simulink model "bh_2dof_compare_models"  (R2017a)
settings: Solver=ode45  StartTime=0.0  StopTime=20  RelTol=1e-5  EnableMultiTasking=on
PreLoadFcn:
  | bh_script_2dof_params
values from neighbouring files (symbols this model uses):
  c1 = 20    [bh_2dof_MATLAB_analysis.m]
  c2 = 50    [bh_2dof_MATLAB_analysis.m]
  c3 = 10    [bh_2dof_MATLAB_analysis.m]
  k1 = 1000    [bh_2dof_MATLAB_analysis.m]
  k2 = 500    [bh_2dof_MATLAB_analysis.m]
  k3 = 100    [bh_2dof_MATLAB_analysis.m]
  m1 = 10    [bh_2dof_MATLAB_analysis.m]
  m2 = 1    [bh_2dof_MATLAB_analysis.m]
undefined symbols (not defined in the file or in its folder): init_x1, init_x1dot, init_x2, init_x2dot
libraries: fl_lib x18, nesl_utility x7
settings Model: Creator=bhorton  LastModifiedBy=bhorton
settings OptimizationCC: LifeSpan=inf
settings DebuggingCC: SFUnexpectedBacktrackingDiag=warning  SFNoUnconditionalDefaultTransitionDiag=warning  SFExecutionAtInitializationDiag=none
settings GRTTargetCC: TargetLangStandard=C89/C90 (ANSI)  GeneratePreprocessorConditionals=Disable all
settings ConfigComp: CovMetricSettings=dw  CovHtmlReporting=on  CovSaveCumulativeToWorkspaceVar=on  CovSaveSingleToWorkspaceVar=on  CovExternalEMLEnable=off

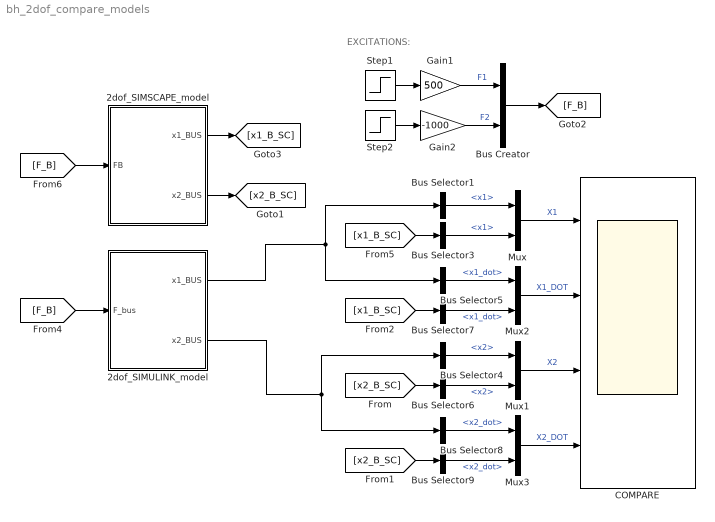
== system bh_2dof_compare_models ==
  note: EXCITATIONS:
  2dof_SIMSCAPE_model : Subsystem
  2dof_SIMULINK_model : Subsystem
  Bus Creator : BusCreator  Inputs=2
  Bus Selector1 : BusSelector  OutputSignals=x1
  Bus Selector3 : BusSelector  OutputSignals=x1
  Bus Selector4 : BusSelector  OutputSignals=x2
  Bus Selector5 : BusSelector  OutputSignals=x1_dot
  Bus Selector6 : BusSelector  OutputSignals=x2
  Bus Selector7 : BusSelector  OutputSignals=x1_dot
  Bus Selector8 : BusSelector  OutputSignals=x2_dot
  Bus Selector9 : BusSelector  OutputSignals=x2_dot
  COMPARE : Scope  NumInputPorts=4
  Gain1 : Gain  Gain=500
  Gain2 : Gain  Gain=-1000
  Mux{,1..3} (4 alike) : Mux  Inputs=2
  Step1 : Step  Time=5  SampleTime=0
  Step2 : Step  Time=10  SampleTime=0
  wires:
  Step1/1 -> Gain1/1
  Gain1/1 -> Bus Creator/1  "F1"
  Step2/1 -> Gain2/1
  Gain2/1 -> Bus Creator/2  "F2"
  Bus Creator/1 -> [F_B]
  [F_B] -> 2dof_SIMSCAPE_model/1(FB)
  [x2_B_SC] -> Bus Selector6/1
  Bus Selector1/1 -> Mux/1  "<x1>"
  [x1_B_SC] -> Bus Selector3/1
  Bus Selector3/1 -> Mux/2  "<x1>"
  Mux/1 -> COMPARE/1  "X1"
  Bus Selector4/1 -> Mux1/1  "<x2>"
  Bus Selector6/1 -> Mux1/2  "<x2>"
  Mux1/1 -> COMPARE/3  "X2"
  2dof_SIMULINK_model/1(x1_BUS) -> Bus Selector5/1, Bus Selector1/1
  Bus Selector5/1 -> Mux2/1  "<x1_dot>"
  [x1_B_SC] -> Bus Selector7/1
  Bus Selector7/1 -> Mux2/2  "<x1_dot>"
  Mux2/1 -> COMPARE/2  "X1_DOT"
  2dof_SIMULINK_model/2(x2_BUS) -> Bus Selector4/1, Bus Selector8/1
  Bus Selector8/1 -> Mux3/1  "<x2_dot>"
  [x2_B_SC] -> Bus Selector9/1
  Bus Selector9/1 -> Mux3/2  "<x2_dot>"
  Mux3/1 -> COMPARE/4  "X2_DOT"
  [F_B] -> 2dof_SIMULINK_model/1(F_bus)
  2dof_SIMSCAPE_model/2(x2_BUS) -> [x2_B_SC]
  2dof_SIMSCAPE_model/1(x1_BUS) -> [x1_B_SC]

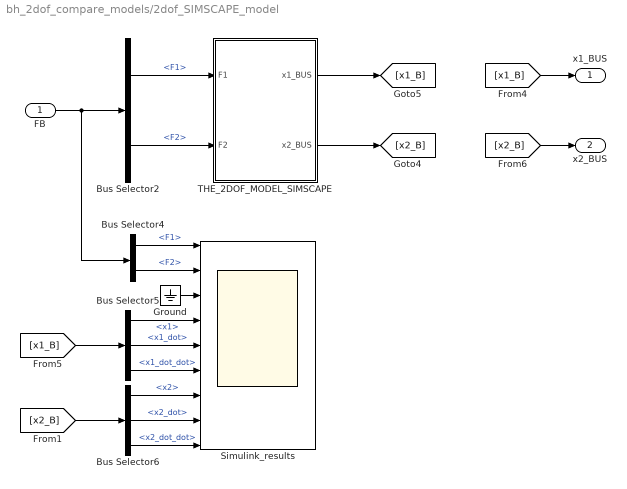
== system bh_2dof_compare_models/2dof_SIMSCAPE_model ==
  FB : Inport
  Bus Selector2 : BusSelector  OutputSignals=F1,F2
  Bus Selector4 : BusSelector  OutputSignals=F1,F2
  Bus Selector5 : BusSelector  OutputSignals=x1,x1_dot,x1_dot_dot
  Bus Selector6 : BusSelector  OutputSignals=x2,x2_dot,x2_dot_dot
  Ground : Ground
  Simulink_results : Scope  NumInputPorts=9
  THE_2DOF_MODEL_SIMSCAPE : Subsystem
  x1_BUS : Outport
  x2_BUS : Outport  Port=2
  wires:
  Bus Selector2/2 -> THE_2DOF_MODEL_SIMSCAPE/2(F2)  "<F2>"
  Bus Selector2/1 -> THE_2DOF_MODEL_SIMSCAPE/1(F1)  "<F1>"
  THE_2DOF_MODEL_SIMSCAPE/1(x1_BUS) -> [x1_B]
  THE_2DOF_MODEL_SIMSCAPE/2(x2_BUS) -> [x2_B]
  [x1_B] -> x1_BUS/1
  [x2_B] -> x2_BUS/1
  FB/1 -> Bus Selector4/1, Bus Selector2/1
  Bus Selector4/1 -> Simulink_results/1  "<F1>"
  Bus Selector4/2 -> Simulink_results/2  "<F2>"
  Ground/1 -> Simulink_results/3
  [x1_B] -> Bus Selector5/1
  Bus Selector5/3 -> Simulink_results/6  "<x1_dot_dot>"
  Bus Selector5/2 -> Simulink_results/5  "<x1_dot>"
  Bus Selector5/1 -> Simulink_results/4  "<x1>"
  Bus Selector6/1 -> Simulink_results/7  "<x2>"
  Bus Selector6/2 -> Simulink_results/8  "<x2_dot>"
  [x2_B] -> Bus Selector6/1
  Bus Selector6/3 -> Simulink_results/9  "<x2_dot_dot>"

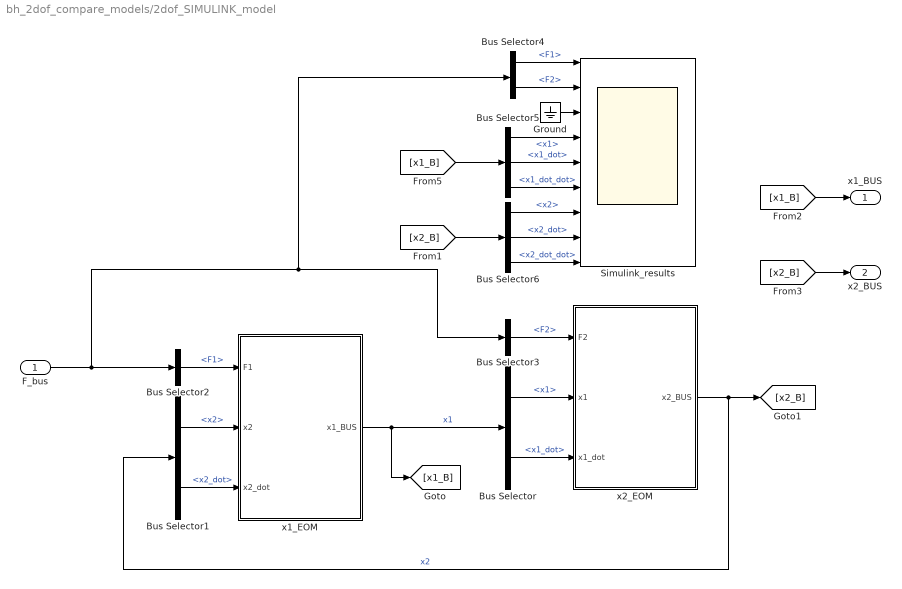
== system bh_2dof_compare_models/2dof_SIMULINK_model ==
  F_bus : Inport
  Bus Selector : BusSelector  OutputSignals=x1,x1_dot
  Bus Selector1 : BusSelector  OutputSignals=x2,x2_dot
  Bus Selector2 : BusSelector  OutputSignals=F1
  Bus Selector3 : BusSelector  OutputSignals=F2
  Bus Selector4 : BusSelector  OutputSignals=F1,F2
  Bus Selector5 : BusSelector  OutputSignals=x1,x1_dot,x1_dot_dot
  Bus Selector6 : BusSelector  OutputSignals=x2,x2_dot,x2_dot_dot
  Ground : Ground
  Simulink_results : Scope  NumInputPorts=9
  x1_EOM : Subsystem
  x2_EOM : Subsystem
  x1_BUS : Outport
  x2_BUS : Outport  Port=2
  wires:
  Bus Selector/2 -> x2_EOM/3(x1_dot)  "<x1_dot>"
  Bus Selector/1 -> x2_EOM/2(x1)  "<x1>"
  Bus Selector1/1 -> x1_EOM/2(x2)  "<x2>"
  Bus Selector1/2 -> x1_EOM/3(x2_dot)  "<x2_dot>"
  x1_EOM/1(x1_BUS) -> [x1_B], Bus Selector/1  "x1"
  x2_EOM/1(x2_BUS) -> Bus Selector1/1, [x2_B]  "x2"
  Bus Selector2/1 -> x1_EOM/1(F1)  "<F1>"
  Bus Selector3/1 -> x2_EOM/1(F2)  "<F2>"
  F_bus/1 -> Bus Selector4/1, Bus Selector3/1, Bus Selector2/1
  Bus Selector4/1 -> Simulink_results/1  "<F1>"
  Bus Selector4/2 -> Simulink_results/2  "<F2>"
  Ground/1 -> Simulink_results/3
  [x1_B] -> Bus Selector5/1
  Bus Selector5/3 -> Simulink_results/6  "<x1_dot_dot>"
  Bus Selector5/2 -> Simulink_results/5  "<x1_dot>"
  Bus Selector5/1 -> Simulink_results/4  "<x1>"
  Bus Selector6/1 -> Simulink_results/7  "<x2>"
  Bus Selector6/2 -> Simulink_results/8  "<x2_dot>"
  Bus Selector6/3 -> Simulink_results/9  "<x2_dot_dot>"
  [x2_B] -> Bus Selector6/1
  [x1_B] -> x1_BUS/1
  [x2_B] -> x2_BUS/1

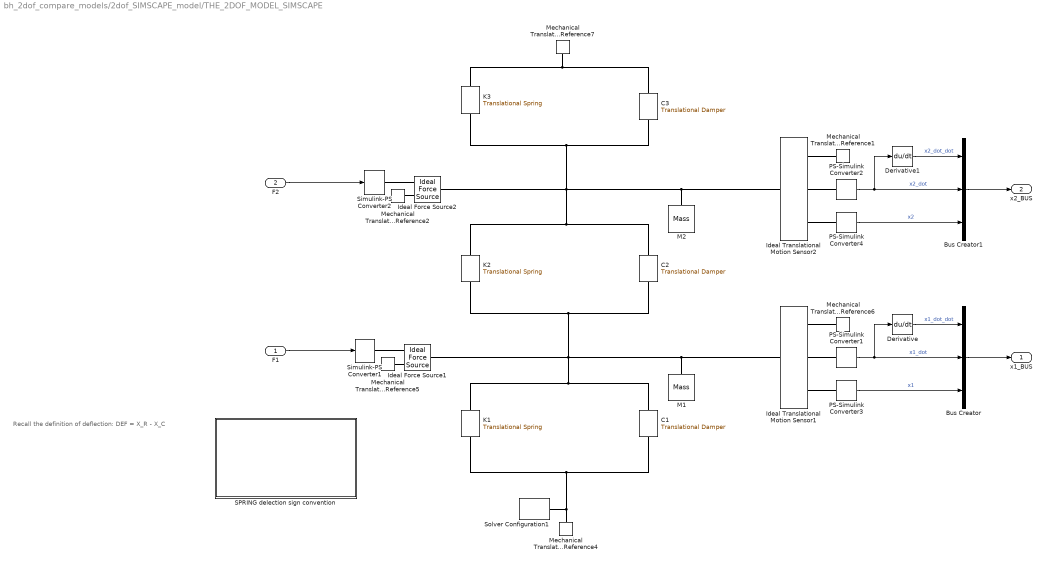
== system bh_2dof_compare_models/2dof_SIMSCAPE_model/THE_2DOF_MODEL_SIMSCAPE ==
  note: Recall the definition of deflection:
      |
      |          DEF = X_R - X_C
  F1 : Inport
  F2 : Inport  Port=2
  Bus Creator : BusCreator  Inputs=3
  Bus Creator1 : BusCreator  Inputs=3
  C1 : fl_lib/Mechanical/Translational Elements/Translational Damper  D=c1 N/(m/s)  v_specify=off  v_priority=None  v=0 m/s  v_nominal_specify=off  v_nominal_unit=m/s  v_nominal_value=1  f_specify=off  f_priority=None  f=0 N  f_nominal_specify=off  f_nominal_unit=N  f_nominal_value=1
      settings: AttributesFormatString=C= %<D>
  C2 : fl_lib/Mechanical/Translational Elements/Translational Damper  D=c2 N/(m/s)  v_specify=off  v_priority=None  v=0 m/s  v_nominal_specify=off  v_nominal_unit=m/s  v_nominal_value=1  f_specify=off  f_priority=None  f=0 N  f_nominal_specify=off  f_nominal_unit=N  f_nominal_value=1
      settings: AttributesFormatString=C= %<D>
  C3 : fl_lib/Mechanical/Translational Elements/Translational Damper  D=c3 N/(m/s)  v_specify=off  v_priority=None  v=0 m/s  v_nominal_specify=off  v_nominal_unit=m/s  v_nominal_value=1  f_specify=off  f_priority=None  f=0 N  f_nominal_specify=off  f_nominal_unit=N  f_nominal_value=1
      settings: AttributesFormatString=C= %<D>
  Derivative : Derivative
  Derivative1 : Derivative
  Ideal Force Source1 : fl_lib/Mechanical/Mechanical Sources/Ideal Force Source
  Ideal Force Source2 : fl_lib/Mechanical/Mechanical Sources/Ideal Force Source
  Ideal Translational Motion Sensor1 : fl_lib/Mechanical/Mechanical Sensors/Ideal Translational Motion Sensor  offset=def_k1.xC m
      settings: AttributesFormatString=OFFSET= %<offset>
  Ideal Translational Motion Sensor2 : fl_lib/Mechanical/Mechanical Sensors/Ideal Translational Motion Sensor  offset=def_k2.xC m
      settings: AttributesFormatString=OFFSET= %<offset>
  K1 : fl_lib/Mechanical/Translational Elements/Translational Spring  spr_rate=k1 N/m  v_specify=off  v_priority=High  v=0 m/s  v_nominal_specify=off  v_nominal_unit=m/s  v_nominal_value=1  f_specify=off  f_priority=None  f=0 N  f_nominal_specify=off  f_nominal_unit=N  f_nominal_value=1  x_specify=on  x_priority=High  x=def_k1.x_def m  x_nominal_specify=off  x_nominal_unit=m  x_nominal_value=1
      settings: AttributesFormatString=|
      | K= %<spr_rate>
      | X_DEF= %<x>
  K2 : fl_lib/Mechanical/Translational Elements/Translational Spring  spr_rate=k2 N/m  v_specify=off  v_priority=High  v=0 m/s  v_nominal_specify=off  v_nominal_unit=m/s  v_nominal_value=1  f_specify=off  f_priority=None  f=0 N  f_nominal_specify=off  f_nominal_unit=N  f_nominal_value=1  x_specify=on  x_priority=High  x=def_k2.x_def m  x_nominal_specify=off  x_nominal_unit=m  x_nominal_value=1
      settings: AttributesFormatString=|
      | K= %<spr_rate>
      | X_DEF= %<x>
  K3 : fl_lib/Mechanical/Translational Elements/Translational Spring  spr_rate=k3 N/m  v_specify=off  v_priority=High  v=0 m/s  v_nominal_specify=off  v_nominal_unit=m/s  v_nominal_value=1  f_specify=off  f_priority=None  f=0 N  f_nominal_specify=off  f_nominal_unit=N  f_nominal_value=1  x_specify=on  x_priority=High  x=def_k3.x_def m  x_nominal_specify=off  x_nominal_unit=m  x_nominal_value=1
      settings: AttributesFormatString=|
      | K= %<spr_rate>
      | X_DEF= %<x>
  M1 : fl_lib/Mechanical/Translational Elements/Mass  mass=m1 kg  v_specify=on  v_priority=High  v=def_k1.vC m/s  v_nominal_specify=off  v_nominal_unit=m/s  v_nominal_value=1  f_specify=off  f_priority=None  f=0 N  f_nominal_specify=off  f_nominal_unit=N  f_nominal_value=1
      settings: AttributesFormatString=|
      | m= %<mass>
      | v = %<v>
  M2 : fl_lib/Mechanical/Translational Elements/Mass  mass=m2 kg  v_specify=on  v_priority=High  v=def_k2.vC m/s  v_nominal_specify=off  v_nominal_unit=m/s  v_nominal_value=1  f_specify=off  f_priority=None  f=0 N  f_nominal_specify=off  f_nominal_unit=N  f_nominal_value=1
      settings: AttributesFormatString=|
      | m= %<mass>
      | v = %<v>
  Mechanical Translational Reference{1..2,4..7} (6 alike) : fl_lib/Mechanical/Translational Elements/Mechanical Translational Reference
  PS-Simulink Converter1 : nesl_utility/PS-Simulink Converter  PhysicalDomain=network_engine_domain  SubClassName=ps_output  LeftPortType=input  RightPortType=output  PseudoPeriodic=off  Frequencies=[]  Unit=m/s  AffineConversion=off
  PS-Simulink Converter2 : nesl_utility/PS-Simulink Converter  PhysicalDomain=network_engine_domain  SubClassName=ps_output  LeftPortType=input  RightPortType=output  PseudoPeriodic=off  Frequencies=[]  Unit=m/s  AffineConversion=off
  PS-Simulink Converter3 : nesl_utility/PS-Simulink Converter  PhysicalDomain=network_engine_domain  SubClassName=ps_output  LeftPortType=input  RightPortType=output  PseudoPeriodic=off  Frequencies=[]  Unit=m  AffineConversion=off
  PS-Simulink Converter4 : nesl_utility/PS-Simulink Converter  PhysicalDomain=network_engine_domain  SubClassName=ps_output  LeftPortType=input  RightPortType=output  PseudoPeriodic=off  Frequencies=[]  Unit=m  AffineConversion=off
  SPRING delection sign convention : Subsystem
  Simulink-PS Converter1 : nesl_utility/Simulink-PS Converter  PhysicalDomain=network_engine_domain  SubClassName=ps_input  LeftPortType=input  RightPortType=output  PseudoPeriodic=off  Frequencies=[]  NoiseDistribution=none  NoiseParameters=[]  Unit=N  AffineConversion=off  FilteringAndDerivatives=zero  SimscapeFilterOrder=1  InputFilterTimeConstant=0.001  UdotUserProvided=1
  Simulink-PS Converter2 : nesl_utility/Simulink-PS Converter  PhysicalDomain=network_engine_domain  SubClassName=ps_input  LeftPortType=input  RightPortType=output  PseudoPeriodic=off  Frequencies=[]  NoiseDistribution=none  NoiseParameters=[]  Unit=N  AffineConversion=off  FilteringAndDerivatives=zero  SimscapeFilterOrder=1  InputFilterTimeConstant=0.001  UdotUserProvided=1
  Solver Configuration1 : nesl_utility/Solver Configuration  PhysicalDomain=network_engine_domain  SubClassName=solver  LeftPortType=input  RightPortType=generic  Accelerate=off  Tones=[]  Harmonics=[]  SimulateNoise=off  Profile=off  UseLocalSampling=off  EnableSwitchedLinearOptims=on  FrequencyDomain=off  UseCCode=off  RelTol=0.001  AbsTol=1e-06  MinStep=1e-09  ToWorkspace=off  RevertToSquareIcSolve=off  NumHomotopyIterations=100  PhasorMode=off  PhasorModeNumHarmonics=1  OverrideAbsTol=off  DoDC=off  ResidualTolerance=1e-09  UseLocalSolver=off  LocalSolverChoice=NE_BACKWARD_EULER_ADVANCER  LocalSolverSampleTime=0.001  DoFixedCost=off  MaxNonlinIter=3  MaxModeIter=2  LinearAlgebra=Sparse  DelaysMemoryBudget=1024  AutomaticFiltering=on  FilteringTimeConstant=0.001
  x1_BUS : Outport
  x2_BUS : Outport  Port=2
  wires:
  F1/1 -> Simulink-PS Converter1/1
  PS-Simulink Converter1/1 -> Bus Creator/2, Derivative/1  "x1_dot"
  Derivative/1 -> Bus Creator/1  "x1_dot_dot"
  PS-Simulink Converter3/1 -> Bus Creator/3  "x1"
  PS-Simulink Converter2/1 -> Bus Creator1/2, Derivative1/1  "x2_dot"
  Derivative1/1 -> Bus Creator1/1  "x2_dot_dot"
  PS-Simulink Converter4/1 -> Bus Creator1/3  "x2"
  F2/1 -> Simulink-PS Converter2/1
  Bus Creator/1 -> x1_BUS/1
  Bus Creator1/1 -> x2_BUS/1
  connections:
  Mechanical Translational Reference4/LConn1 -- Solver Configuration1/RConn1 -- K1/LConn1 -- C1/LConn1
  C1/RConn1 -- K1/RConn1 -- Ideal Translational Motion Sensor1/LConn1 -- M1/LConn1 -- Ideal Force Source1/LConn1 -- C2/LConn1 -- K2/LConn1
  Ideal Force Source2/LConn1 -- M2/LConn1 -- Ideal Translational Motion Sensor2/LConn1 -- K2/RConn1 -- C2/RConn1 -- C3/LConn1 -- K3/LConn1
  Mechanical Translational Reference7/LConn1 -- C3/RConn1 -- K3/RConn1
  Simulink-PS Converter2/RConn1 -- Ideal Force Source2/RConn1
  Mechanical Translational Reference2/LConn1 -- Ideal Force Source2/RConn2
  PS-Simulink Converter2/LConn1 -- Ideal Translational Motion Sensor2/RConn2
  Mechanical Translational Reference1/LConn1 -- Ideal Translational Motion Sensor2/RConn1
  Ideal Translational Motion Sensor2/RConn3 -- PS-Simulink Converter4/LConn1
  Mechanical Translational Reference6/LConn1 -- Ideal Translational Motion Sensor1/RConn1
  PS-Simulink Converter1/LConn1 -- Ideal Translational Motion Sensor1/RConn2
  Mechanical Translational Reference5/LConn1 -- Ideal Force Source1/RConn2
  Ideal Translational Motion Sensor1/RConn3 -- PS-Simulink Converter3/LConn1
  Simulink-PS Converter1/RConn1 -- Ideal Force Source1/RConn1

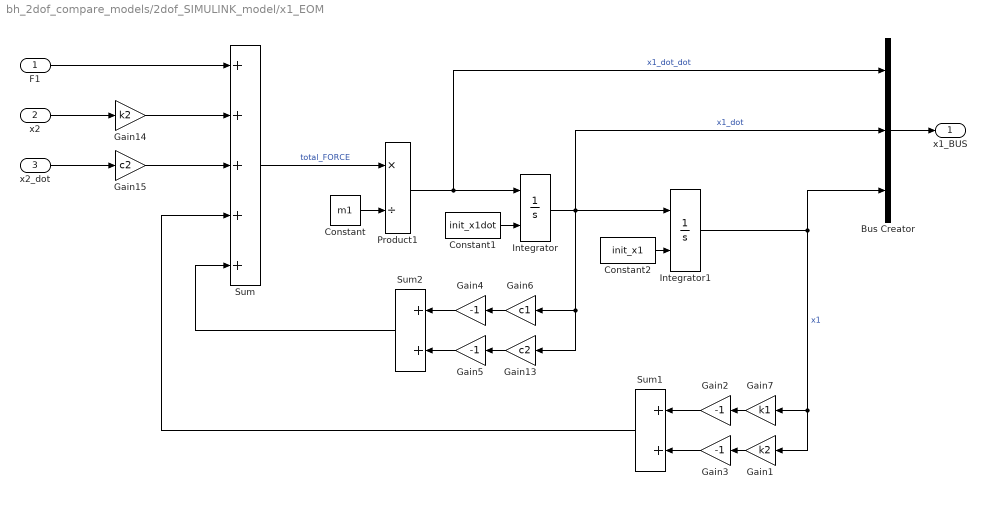
== system bh_2dof_compare_models/2dof_SIMULINK_model/x1_EOM ==
  F1 : Inport
  x2 : Inport  Port=2
  x2_dot : Inport  Port=3
  Bus Creator : BusCreator  Inputs=3
  Constant : Constant  Value=m1
  Constant1 : Constant  Value=init_x1dot
  Constant2 : Constant  Value=init_x1
  Gain1 : Gain  Gain=k2
  Gain13 : Gain  Gain=c2
  Gain14 : Gain  Gain=k2
  Gain15 : Gain  Gain=c2
  Gain{2..5} (4 alike) : Gain  Gain=-1
  Gain6 : Gain  Gain=c1
  Gain7 : Gain  Gain=k1
  Integrator : Integrator  InitialConditionSource=external
  Integrator1 : Integrator  InitialConditionSource=external
  Product1 : Product  Inputs=*/
  Sum : Sum  Inputs=+|+|+|+|+
  Sum1 : Sum  Inputs=2
  Sum2 : Sum  Inputs=2
  x1_BUS : Outport
  wires:
  F1/1 -> Sum/1
  Gain3/1 -> Sum1/2
  Gain4/1 -> Sum2/1
  Gain14/1 -> Sum/2
  Gain6/1 -> Gain4/1
  x2/1 -> Gain14/1
  Gain2/1 -> Sum1/1
  Sum2/1 -> Sum/5
  Sum1/1 -> Sum/4
  x2_dot/1 -> Gain15/1
  Gain15/1 -> Sum/3
  Constant/1 -> Product1/2
  Sum/1 -> Product1/1  "total_FORCE"
  Integrator/1 -> Bus Creator/2, Integrator1/1, Gain13/1, Gain6/1  "x1_dot"
  Product1/1 -> Bus Creator/1, Integrator/1  "x1_dot_dot"
  Integrator1/1 -> Bus Creator/3, Gain7/1, Gain1/1  "x1"
  Bus Creator/1 -> x1_BUS/1
  Gain7/1 -> Gain2/1
  Gain1/1 -> Gain3/1
  Gain5/1 -> Sum2/2
  Gain13/1 -> Gain5/1
  Constant1/1 -> Integrator/2
  Constant2/1 -> Integrator1/2

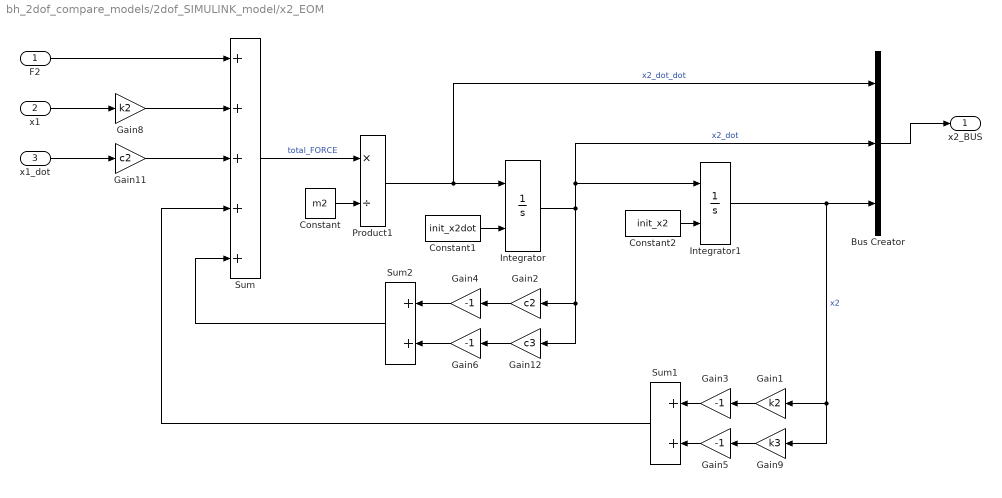
== system bh_2dof_compare_models/2dof_SIMULINK_model/x2_EOM ==
  F2 : Inport
  x1 : Inport  Port=2
  x1_dot : Inport  Port=3
  Bus Creator : BusCreator  Inputs=3
  Constant : Constant  Value=m2
  Constant1 : Constant  Value=init_x2dot
  Constant2 : Constant  Value=init_x2
  Gain1 : Gain  Gain=k2
  Gain11 : Gain  Gain=c2
  Gain12 : Gain  Gain=c3
  Gain2 : Gain  Gain=c2
  Gain{3..6} (4 alike) : Gain  Gain=-1
  Gain8 : Gain  Gain=k2
  Gain9 : Gain  Gain=k3
  Integrator : Integrator  InitialConditionSource=external
  Integrator1 : Integrator  InitialConditionSource=external
  Product1 : Product  Inputs=*/
  Sum : Sum  Inputs=+|+|+|+|+
  Sum1 : Sum  Inputs=2
  Sum2 : Sum  Inputs=2
  x2_BUS : Outport
  wires:
  F2/1 -> Sum/1
  Gain9/1 -> Gain5/1
  Gain4/1 -> Sum2/1
  Gain8/1 -> Sum/2
  x1/1 -> Gain8/1
  Gain12/1 -> Gain6/1
  Sum2/1 -> Sum/5
  Sum1/1 -> Sum/4
  x1_dot/1 -> Gain11/1
  Gain11/1 -> Sum/3
  Constant/1 -> Product1/2
  Sum/1 -> Product1/1  "total_FORCE"
  Integrator/1 -> Integrator1/1, Bus Creator/2, Gain12/1, Gain2/1  "x2_dot"
  Product1/1 -> Bus Creator/1, Integrator/1  "x2_dot_dot"
  Integrator1/1 -> Bus Creator/3, Gain9/1, Gain1/1  "x2"
  Gain3/1 -> Sum1/1
  Gain1/1 -> Gain3/1
  Gain2/1 -> Gain4/1
  Bus Creator/1 -> x2_BUS/1
  Gain5/1 -> Sum1/2
  Gain6/1 -> Sum2/2
  Constant1/1 -> Integrator/2
  Constant2/1 -> Integrator1/2

== system bh_2dof_compare_models/2dof_SIMSCAPE_model/THE_2DOF_MODEL_SIMSCAPE/SPRING delection sign convention ==
  note: deflection is NEGATIVE (-)
  note: deflection is POSITIVE (+)
